simulink model "sy408022311"  (R2022b)
settings: Solver=VariableStepAuto  StartTime=0.0  StopTime=7  RelTol=1e-3
settings Model: Creator=ASUS  LastModifiedBy=ASUS

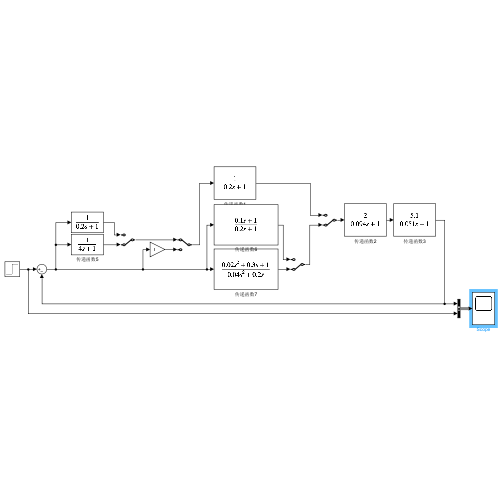
[thumbnail: Simulink's stored preview of the top-level diagram]
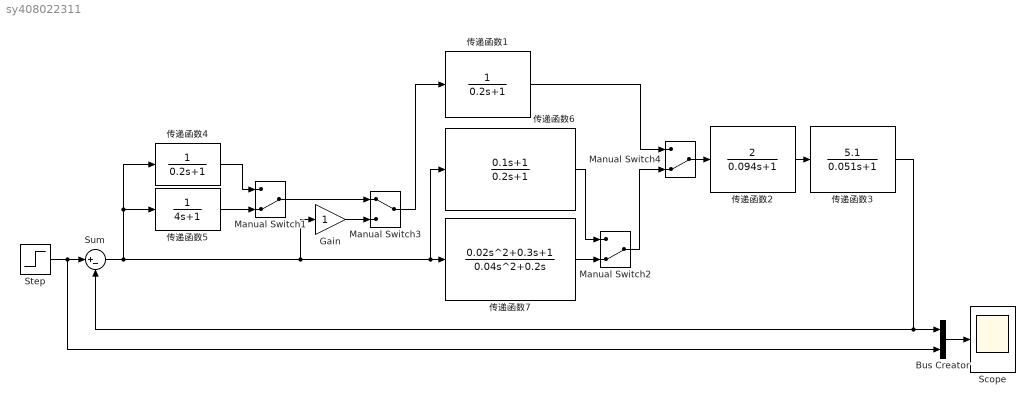
== system sy408022311 ==
  Bus Creator : BusCreator  Inputs=2
  Gain : Gain
  Manual Switch1 : ManualSwitch  CurrentSetting=0
  Manual Switch2 : ManualSwitch  CurrentSetting=0
  Manual Switch3 : ManualSwitch
  Manual Switch4 : ManualSwitch  CurrentSetting=0
  Scope : Scope
  Step : Step  After=3  SampleTime=0
  Sum : Sum  Inputs=|+-
  传递函数1 : TransferFcn  Denominator=[0.2 1]
  传递函数2 : TransferFcn  Numerator=[2]  Denominator=[0.094 1]
  传递函数3 : TransferFcn  Numerator=[5.1]  Denominator=[0.051 1]
  传递函数4 : TransferFcn  Denominator=[0.2 1]
  传递函数5 : TransferFcn  Denominator=[4 1]
  传递函数6 : TransferFcn  Numerator=[0.1 1]  Denominator=[0.2 1]
  传递函数7 : TransferFcn  Numerator=[0.02 0.3 1]  Denominator=[0.04 0.2 0]
  wires:
  传递函数3/1 -> Sum/2, Bus Creator/1
  Step/1 -> Bus Creator/2, Sum/1
  Bus Creator/1 -> Scope/1
  传递函数2/1 -> 传递函数3/1
  Manual Switch3/1 -> 传递函数1/1
  Manual Switch1/1 -> Manual Switch3/1
  Gain/1 -> Manual Switch3/2
  传递函数4/1 -> Manual Switch1/1
  传递函数5/1 -> Manual Switch1/2
  Sum/1 -> 传递函数6/1, 传递函数7/1, Gain/1, 传递函数4/1, 传递函数5/1
  传递函数7/1 -> Manual Switch2/2
  传递函数1/1 -> Manual Switch4/1
  Manual Switch4/1 -> 传递函数2/1
  Manual Switch2/1 -> Manual Switch4/2
  传递函数6/1 -> Manual Switch2/1
